simulink model "E040S0_S2_guard_shed_iqcot_20260629"  (R2024b)
settings: Solver=VariableStepAuto  StartTime=0.0  StopTime=0.52e-3  MaxStep=5e-9  RelTol=1e-3
undefined symbols (not defined in the file): A_init, A_lower, A_upper, Cout, DCR_L1, DCR_L2, DCR_L3, DCR_L4, E040_Calibration_Enable, E040_Current_Deadband, E040_Current_Limit_A, E040_Dwell_Time, E040_Fallback_K_T, E040_I_Shed_Low, E040_IL_Sense_Gain1, E040_IL_Sense_Gain2, E040_IL_Sense_Gain3, E040_IL_Sense_Gain4, E040_K_T, E040_LoadStep_Time, E040_Min_Scale, E040_Order_Relock_Window, E040_Post_Reentry_Shed_Delay, E040_Residual_Current_Threshold, E040_Sense_Confidence, E040_Severe_Overshoot_Band, E040_T_Trim_Max, E040_TonDiff_Enable, E040_V_Error_Budget, E040_V_Error_Hard_Limit, E040_Variant_Mode, E040_Vref, ESR_C, IdealIQCOT_Enable, IL_adc_counts_per_A, IL_pk_limit_adc_neg, IL_pk_limit_adc_pos, Iload_final, Iload_initial, Iph, Iqcot_enable, kappa_cmd, Kiqcot, Kvc_iqcot, L, Lambda0_iqcot, Lambda_m2, rho_cmd, Ri_iqcot, t_load_step, Tblank, Tdead, Tiqcot_leak, Toff_min, Ton_cmd, Ton_iq_max, Ton_iq_min, Ts_ctrl, Tslot, Tss ... (+6)
libraries: simulink x29, spsCurrentMeasurementLib x8, spsMosfetLib x8, spsSeriesRLCBranchLib x5, spsVoltageMeasurementLib x5, spsDCVoltageSourceLib x4, spsControlledCurrentSourceLib x1, spsGroundLib x1, spspowerguiLib x1
(part 1 of 2)
settings Model: Creator=zengruize  LastModifiedBy=zengruize

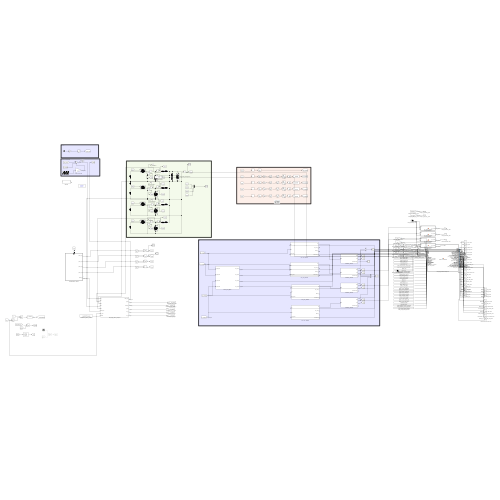
[thumbnail: Simulink's stored preview of the top-level diagram]
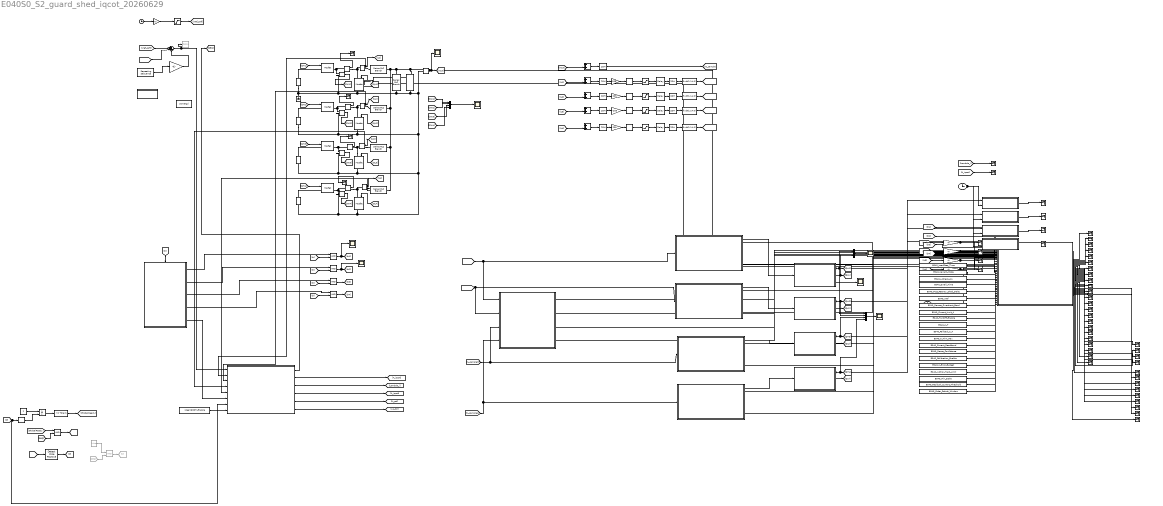
== system E040S0_S2_guard_shed_iqcot_20260629 ==
  note: cot
  note: 输出电压误差比较器
  note: 功率级
  note: 软启动
  note: 采样
  Add{,1..4} (5 alike) : Sum
  Bus Creator : BusCreator  Inputs=4
  Bus Creator1 : BusCreator  Inputs=2
  Bus Creator2 : BusCreator  Inputs=4
  COT_Cell_1Phase1 : Subsystem
  COT_Cell_1Phase2 : Subsystem
  COT_Cell_1Phase3 : Subsystem
  COT_Cell_1Phase4 : Subsystem
  Clock : Clock
  Compare To Constant : simulink/Logic and Bit Operations/Compare To Constant  relop=>=  const=Tblank  OutDataTypeStr=boolean
  Constant : Constant
  Current Measurement{,1..3} (4 alike) : spsCurrentMeasurementLib/Current Measurement  PhasorSimulation=off  OutputType=Complex  PSBequivalent=0
  DC Voltage Source{,1..3} (4 alike) : spsDCVoltageSourceLib/DC Voltage Source  Amplitude=Vin  Measurements=None
  Data Type Conversion{,2..4} (4 alike) : DataTypeConversion  OutDataTypeStr=fixdt(1,14,0)  SaturateOnIntegerOverflow=off  RndMeth=Floor
  Detect Rise Positive : simulink/Logic and Bit Operations/Detect Rise Positive  vinit=0  OutDataTypeStr=boolean
  E040_Calibration_Enable : Constant  Value=E040_Calibration_Enable
  E040_Current_Deadband : Constant  Value=E040_Current_Deadband
  E040_Current_Limit_A : Constant  Value=E040_Current_Limit_A
  E040_Dwell_Time : Constant  Value=E040_Dwell_Time
  E040_Fallback_K_T : Constant  Value=E040_Fallback_K_T
  E040_IL_Sense_Gain_Block1 : Gain  Gain=E040_IL_Sense_Gain1
  E040_IL_Sense_Gain_Block2 : Gain  Gain=E040_IL_Sense_Gain2
  E040_IL_Sense_Gain_Block3 : Gain  Gain=E040_IL_Sense_Gain3
  E040_IL_Sense_Gain_Block4 : Gain  Gain=E040_IL_Sense_Gain4
  E040_IL_Sense_Term{1..4} (4 alike) : Terminator
  E040_I_Shed_Low : Constant  Value=E040_I_Shed_Low
  E040_K_T : Constant  Value=E040_K_T
  E040_LoadCurrentStep : Step  Time=t_load_step  Before=Iload_initial  After=Iload_final  SampleTime=0
  E040_LoadStep_Time : Constant  Value=E040_LoadStep_Time
  E040_Load_Current_Source : spsControlledCurrentSourceLib/Controlled Current Source  Initialize=on  Source_Type=DC  Amplitude=0  Phase=0  Frequency=0  Measurements=None
  E040_Log_Lambda_i_Term : Terminator
  E040_Log_area_int_i_Term : Terminator
  E040_Min_Scale : Constant  Value=E040_Min_Scale
  E040_N_active_Term : Terminator
  E040_Order_Relock_Window : Constant  Value=E040_Order_Relock_Window
  E040_Post_Reentry_Shed_Delay : Constant  Value=E040_Post_Reentry_Shed_Delay
  E040_REQ_accept1_Term : Terminator
  E040_REQ_accept2_Term : Terminator
  E040_REQ_accept3_Term : Terminator
  E040_REQ_accept4_Term : Terminator
  E040_REQ_reject_reason_Term : Terminator
  E040_Residual_Current_Threshold : Constant  Value=E040_Residual_Current_Threshold
  E040_S0_ShedPhaseSupervisor : MATLAB Function  TreatAsAtomicUnit=on
  E040_S0_Supervisor_Clock : Clock
  E040_Sense_Confidence : Constant  Value=E040_Sense_Confidence
  E040_Severe_Overshoot_Band : Constant  Value=E040_Severe_Overshoot_Band
  E040_T_Trim_Max : Constant  Value=E040_T_Trim_Max
  E040_TonActual1 : MATLAB Function  TreatAsAtomicUnit=on  SystemSampleTime=Ts_ctrl
  E040_TonActual1_Term : Terminator
  E040_TonActual2 : MATLAB Function  TreatAsAtomicUnit=on  SystemSampleTime=Ts_ctrl
  E040_TonActual2_Term : Terminator
  E040_TonActual3 : MATLAB Function  TreatAsAtomicUnit=on  SystemSampleTime=Ts_ctrl
  E040_TonActual3_Term : Terminator
  E040_TonActual4 : MATLAB Function  TreatAsAtomicUnit=on  SystemSampleTime=Ts_ctrl
  E040_TonActual4_Term : Terminator
  E040_TonActual_Clock : Clock
  E040_TonDiff_Enable : Constant  Value=E040_TonDiff_Enable
  E040_Ton_trim1_Term : Terminator
  E040_Ton_trim2_Term : Terminator
  E040_Ton_trim3_Term : Terminator
  E040_Ton_trim4_Term : Terminator
  E040_V_Error_Budget : Constant  Value=E040_V_Error_Budget
  E040_V_Error_Hard_Limit : Constant  Value=E040_V_Error_Hard_Limit
  E040_Variant_Mode : Constant  Value=E040_Variant_Mode
  E040_Vref : Constant  Value=E040_Vref
  E040_a_S_enable_after_shed_Term : Terminator
  E040_a_S_mode_Term : Terminator
  E040_active_phase_set_Term : Terminator
  E040_balance_recovery_state_Term : Terminator
  E040_calibration_enable_Term : Terminator
  E040_current_limit_hit_Term : Terminator
  E040_dwell_timer_Term : Terminator
  E040_fallback_count_Term : Terminator
  E040_guard_clamp_count_Term : Terminator
  E040_logical_slot_Term : Terminator
  E040_order_relock_state_Term : Terminator
  E040_order_relock_window_done_Term : Terminator
  E040_phase_add_request_Term : Terminator
  E040_phase_order_error_rate_window_Term : Terminator
  E040_phase_shed_accept_Term : Terminator
  E040_phase_shed_reject_Term : Terminator
  E040_phase_shed_reject_reason_Term : Terminator
  E040_phase_shed_request_Term : Terminator
  E040_physical_phase_selected_Term : Terminator
  E040_post_reentry_shed_delay_timer_Term : Terminator
  E040_protect_state_Term : Terminator
  E040_reentry_state_Term : Terminator
  E040_residual_current_check_Term : Terminator
  E040_residual_current_i_Term : Terminator
  E040_residual_current_threshold_Term : Terminator
  E040_sense_confidence_Term : Terminator
  E040_shed_lockout_state_Term : Terminator
  E040_shed_state_Term : Terminator
  From31 : From  Commented=on  GotoTag=REQ
  Gain : Gain  Gain=Vo_ref / Tss
  Gain11 : Gain  Gain=205
  Gain12 : Gain  Gain=-205
  Gain13 : Gain  Gain=205
  Gain9 : Gain  Gain=-205
  GateDriver_1Phase1 : Subsystem
  GateDriver_1Phase2 : Subsystem
  GateDriver_1Phase3 : Subsystem
  GateDriver_1Phase4 : Subsystem
  Goto26 : Goto  Commented=on  GotoTag=tr
  Ground : spsGroundLib/Ground  LConnTagsString=a
  IHS_Terminator{1..4} (4 alike) : Terminator
  IL_Measurement{1..4} (4 alike) : spsCurrentMeasurementLib/Current Measurement  PhasorSimulation=off  OutputType=Complex  PSBequivalent=0
  IQCOT_Ton_Adapter : Subsystem
  IdealIQCOT_Enable_Constant : Constant  Value=IdealIQCOT_Enable
  Ideal_Digital_IQCOT_Request : Subsystem
  Integrator : Integrator  ExternalReset=rising
  Logical Operator{,1..4} (5 alike) : Logic  AllPortsSameDT=off  OutDataTypeStr=boolean
  Logical Operator5 : Logic  Commented=on  AllPortsSameDT=off  OutDataTypeStr=boolean
  Memory : Memory
  Mosfet{,1..3} (4 alike) : spsMosfetLib/Mosfet  Ron=Ron_HS  Lon=0  Rd=Rd_body  Vfd=Vfd_body  IC=0  Rs=Rs_snubber  Cs=Cs_snubber  Measurements=on
  Mosfet{4..7} (4 alike) : spsMosfetLib/Mosfet  Ron=Ron_LS  Lon=0  Rd=Rd_body  Vfd=Vfd_body  IC=0  Rs=Rs_snubber  Cs=Cs_snubber  Measurements=on
  OnDelay : Subsystem
  PhaseScheduler_4Phase : Subsystem  TreatAsAtomicUnit=on
  Pulse Generator : DiscretePulseGenerator  Commented=on  PulseType=Time based  Period=Tblank  PulseWidth=5
  Quantizer{1..4} (4 alike) : Quantizer  QuantizationInterval=1
  Relay : Relay  Commented=through  OnSwitchValue=Vhys/2  OffSwitchValue=-Vhys/2
  Saturation{,1,3..4} (4 alike) : Saturate  UpperLimit=8191  LowerLimit=-8191
  Saturation2 : Saturate  UpperLimit=Vo_ref  LowerLimit=0
  Scope{,1..6} (7 alike) : Scope
  Series RLC Branch : spsSeriesRLCBranchLib/Series RLC Branch  LConnTagsString=__new0  RConnTagsString=__new0  BranchType=RL  Resistance=DCR_L1  Inductance=L  SetiL0=off  InitialCurrent=0  Capacitance=1e-6  Setx0=off  InitialVoltage=0  Measurements=None
  Series RLC Branch1 : spsSeriesRLCBranchLib/Series RLC Branch  LConnTagsString=__new0  RConnTagsString=__new0  BranchType=RL  Resistance=DCR_L2  Inductance=L  SetiL0=off  InitialCurrent=0  Capacitance=1e-6  Setx0=off  InitialVoltage=0  Measurements=None
  Series RLC Branch2 : spsSeriesRLCBranchLib/Series RLC Branch  LConnTagsString=__new0  RConnTagsString=__new0  BranchType=RL  Resistance=DCR_L3  Inductance=L  SetiL0=off  InitialCurrent=0  Capacitance=1e-6  Setx0=off  InitialVoltage=0  Measurements=None
  Series RLC Branch3 : spsSeriesRLCBranchLib/Series RLC Branch  LConnTagsString=__new0  RConnTagsString=__new0  BranchType=RL  Resistance=DCR_L4  Inductance=L  SetiL0=off  InitialCurrent=0  Capacitance=1e-6  Setx0=off  InitialVoltage=0  Measurements=None
  Series RLC Branch4 : spsSeriesRLCBranchLib/Series RLC Branch  LConnTagsString=__new0  RConnTagsString=__new0  BranchType=RC  Resistance=ESR_C  Inductance=1e-3  SetiL0=off  InitialCurrent=0  Capacitance=Cout  Setx0=on  InitialVoltage=Vo_ref  Measurements=None
  Sum : Sum  Inputs=|+--
  Transport Delay{1..4} (4 alike) : TransportDelay  DelayTime=5/25000000
  VCOT_Ramp_Gain : Gain  Gain=Vcot_ramp_enable * Vcot_ramp_amp
  VCOT_Ramp_Unit : simulink/Sources/Repeating Sequence  rep_seq_t=[0 Tslot]  rep_seq_y=[0 1]
  Voltage Measurement{,1..4} (5 alike) : spsVoltageMeasurementLib/Voltage Measurement  PhasorSimulation=off  OutputType=Complex  PSBequivalent=0
  Zero-Order Hold{1..4,19..23} (9 alike) : ZeroOrderHold  SampleTime=1/25000000
  powergui : spspowerguiLib/powergui  Priority=1  SimulationMode=Discrete  SampleTime=2e-9  frequency=60  Iterations=50  frequencyindice=0  Pbase=100e6  ErrMax=1e-4  UnitsV=kV  UnitsW=MW  buscounter=0  FunctionMessages=off  echomessages=off  EnableUseOfTLC=off  CurrentSourceSwitches=off  DisableSnubberDevices=off  DisableRonSwitches=off  DisableVfSwitches=off  DisplayEquations=off  AutomaticDiscreteSolvers=off  SolverType=Tustin/Backward Euler (TBE)  Interpol=off  ExternalGateDelay=off  methode=off  Ts=100  x0status=blocks  SPID=on  SwTol=0  HookPort=off  NonlinearTolerance=1e-4  nMaxIteration=100  ContinueOnMaxIteration=off  RestoreLinks=warning  ResistiveCurrentMeasurement=off  Frange=[0:2:500]  Ylog=off  Xlog=on  ShowGrid=off  save=off  variable=ZData  structure=0  ZoomFFT=off  StartTime=0.0  cycles=1  DisplayStyle=1  fundamental=60  FreqAxis=off  MaxFrequency=1000  frequencyindicesteady=1  RmsSteady=1  display=off
  wires:
  [QH1] -> Mosfet/1
  [QH4] -> Mosfet3/1
  [QH2] -> Mosfet1/1
  [QH3] -> Mosfet2/1
  [QL1] -> Mosfet4/1
  [QL2] -> Mosfet5/1
  [QL3] -> Mosfet6/1
  [QL4] -> Mosfet7/1
  Voltage Measurement2/1 -> [SW2]  "SW2"
  Voltage Measurement3/1 -> [SW3]  "SW3"
  Voltage Measurement1/1 -> [SW1]  "SW1"
  Voltage Measurement4/1 -> [SW4]  "SW4"
  GateDriver_1Phase1/1(QHi) -> Bus Creator1/1, [QH1], Bus Creator2/1, E040_TonActual1/1(qh)  "QH1"
  GateDriver_1Phase2/1(QHi) -> Bus Creator2/2, [QH2], E040_TonActual2/1(qh)  "QH2"
  GateDriver_1Phase3/1(QHi) -> Bus Creator2/3, [QH3], E040_TonActual3/1(qh)  "QH3"
  GateDriver_1Phase4/1(QHi) -> Bus Creator2/4, [QH4], E040_TonActual4/1(qh)  "QH4"
  GateDriver_1Phase1/2(QLi) -> Bus Creator1/2, [QL1]  "QL1"
  GateDriver_1Phase2/2(QLi) -> [QL2]  "QL2"
  GateDriver_1Phase3/2(QLi) -> [QL3]  "QL3"
  GateDriver_1Phase4/2(QLi) -> [QL4]  "QL4"
  COT_Cell_1Phase1/1(Qi) -> GateDriver_1Phase1/1(Qi)
  COT_Cell_1Phase2/1(Qi) -> GateDriver_1Phase2/1(Qi)
  COT_Cell_1Phase3/1(Qi) -> GateDriver_1Phase3/1(Qi)
  COT_Cell_1Phase4/1(Qi) -> GateDriver_1Phase4/1(Qi)
  GateDriver_1Phase1/3(ShootThrough_i) -> Scope1/1
  Bus Creator/1 -> Scope2/1
  [SW1] -> Bus Creator/1
  [SW2] -> Bus Creator/2
  [SW3] -> Bus Creator/3
  [SW4] -> Bus Creator/4
  Bus Creator1/1 -> Scope3/1
  Saturation2/1 -> [Vref_soft]
  Gain/1 -> Saturation2/1
  Clock/1 -> Gain/1
  Voltage Measurement/1 -> Scope/1, [Vout], E040_S0_ShedPhaseSupervisor/13(vout)  "Vout"
  [Vref_soft] -> Sum/1
  [Vo_sample] -> Sum/2
  Sum/1 -> Ideal_Digital_IQCOT_Request/1(e_v), Relay/1  "e_v"
  Constant/1 -> Integrator/1
  Integrator/1 -> Compare To Constant/1
  Compare To Constant/1 -> [GlobalReady]  "Allow"
  [GlobalReady] -> Logical Operator/1
  [REQ] -> Logical Operator/2
  Logical Operator/1 -> [Allow]
  [Allow] -> Detect Rise Positive/1
  Detect Rise Positive/1 -> [tr]
  [tr] -> PhaseScheduler_4Phase/Trigger  "tr"
  PhaseScheduler_4Phase/1(phase_en1) -> Logical Operator1/1
  [tr] -> Logical Operator1/2
  PhaseScheduler_4Phase/2(phase_en2) -> Logical Operator2/1
  [tr] -> Logical Operator2/2
  PhaseScheduler_4Phase/3(phase_en3) -> Logical Operator3/1
  [tr] -> Logical Operator3/2
  PhaseScheduler_4Phase/4(phase_en4) -> Logical Operator4/1
  [tr] -> Logical Operator4/2
  Logical Operator1/1 -> Scope4/1, [tr1]  "tr1"
  Logical Operator2/1 -> Scope5/1, [tr2]  "tr2"
  Logical Operator3/1 -> [tr3]  "tr3"
  Logical Operator4/1 -> [tr4]  "tr4"
  [IL_sample1] -> COT_Cell_1Phase1/2(ILi), IQCOT_Ton_Adapter/1(IL_sample1)  "IL_sample1"
  [IL_sample2] -> IQCOT_Ton_Adapter/2(IL_sample2), COT_Cell_1Phase2/2(ILi)  "IL_sample2"
  [IL_sample3] -> IQCOT_Ton_Adapter/3(IL_sample3), COT_Cell_1Phase3/2(ILi)  "IL_sample3"
  [IL_sample4] -> IQCOT_Ton_Adapter/4(IL_sample4), COT_Cell_1Phase4/2(ILi)  "IL_sample4"
  [tr] -> Memory/1, Ideal_Digital_IQCOT_Request/7(tr_reset)  "tr_reset"
  Memory/1 -> Integrator/2
  Logical Operator5/1 -> Goto26/1
  Pulse Generator/1 -> Logical Operator5/1
  From31/1 -> Logical Operator5/2
  Bus Creator2/1 -> Scope6/1
  IL_Measurement1/1 -> [IL1], Ideal_Digital_IQCOT_Request/2(IL1)  "IL1"
  IL_Measurement2/1 -> [IL2], Ideal_Digital_IQCOT_Request/3(IL2)  "IL2"
  IL_Measurement3/1 -> [IL3], Ideal_Digital_IQCOT_Request/4(IL3)  "IL3"
  IL_Measurement4/1 -> [IL4], Ideal_Digital_IQCOT_Request/5(IL4)  "IL4"
  Current Measurement/1 -> IHS_Terminator1/1
  Current Measurement1/1 -> IHS_Terminator2/1
  Current Measurement2/1 -> IHS_Terminator3/1
  Current Measurement3/1 -> IHS_Terminator4/1
  Zero-Order Hold23/1 -> Gain13/1
  Zero-Order Hold20/1 -> Gain9/1
  Zero-Order Hold3/1 -> Data Type Conversion3/1
  Zero-Order Hold4/1 -> Data Type Conversion2/1
  Saturation4/1 -> Transport Delay4/1
  Zero-Order Hold1/1 -> Data Type Conversion/1
  [IL3] -> Add3/2
  Add3/1 -> Zero-Order Hold22/1
  Quantizer1/1 -> Saturation/1
  Quantizer4/1 -> Saturation4/1
  Gain12/1 -> Quantizer3/1
  [IL4] -> Add4/2
  Add/1 -> Zero-Order Hold19/1
  Data Type Conversion/1 -> [IL_sample1]
  Data Type Conversion2/1 -> [IL_sample4]
  Add4/1 -> Zero-Order Hold23/1
  Transport Delay3/1 -> Zero-Order Hold3/1
  Saturation3/1 -> Transport Delay3/1
  Add1/1 -> Zero-Order Hold20/1
  [IL1] -> Add1/2
  Transport Delay4/1 -> Zero-Order Hold4/1
  Zero-Order Hold21/1 -> Gain11/1
  Data Type Conversion3/1 -> [IL_sample3]
  Gain9/1 -> Quantizer1/1
  Gain11/1 -> Quantizer2/1
  Saturation/1 -> Transport Delay1/1
  [IL2] -> Add2/2
  Transport Delay2/1 -> Zero-Order Hold2/1
  Zero-Order Hold19/1 -> [Vo_sample]
  Gain13/1 -> Quantizer4/1
  Quantizer3/1 -> Saturation3/1
  Data Type Conversion4/1 -> [IL_sample2]
  Zero-Order Hold2/1 -> Data Type Conversion4/1
  Add2/1 -> Zero-Order Hold21/1
  Transport Delay1/1 -> Zero-Order Hold1/1
  [Vout] -> Add/2
  Saturation1/1 -> Transport Delay2/1
  Zero-Order Hold22/1 -> Gain12/1
  Quantizer2/1 -> Saturation1/1
  VCOT_Ramp_Unit/1 -> VCOT_Ramp_Gain/1
  VCOT_Ramp_Gain/1 -> Sum/3  "Vcot_ramp"
  PhaseScheduler_4Phase/5(phase_idx) -> Ideal_Digital_IQCOT_Request/6(phase_idx)  "phase_idx"
  IdealIQCOT_Enable_Constant/1 -> Ideal_Digital_IQCOT_Request/8(enable)
  Ideal_Digital_IQCOT_Request/1(REQ_iqcot) -> [REQ]  "REQ_iqcot"
  Ideal_Digital_IQCOT_Request/2(A_iqcot) -> [A_iqcot]  "A_iqcot"
  Ideal_Digital_IQCOT_Request/3(Lambda_i) -> [Lambda_i]  "Lambda_i"
  Ideal_Digital_IQCOT_Request/4(h_iqcot) -> [h_iqcot]  "h_iqcot"
  Ideal_Digital_IQCOT_Request/5(IL_sel) -> [IL_sel]  "IL_sel"
  Ideal_Digital_IQCOT_Request/6(vc_ctrl) -> [vc_ctrl]  "vc_ctrl"
  E040_LoadCurrentStep/1 -> E040_Load_Current_Source/1, E040_S0_ShedPhaseSupervisor/14(iload)  "Iload"
  [IL1] -> E040_IL_Sense_Gain_Block1/1
  E040_IL_Sense_Gain_Block1/1 -> E040_IL_Sense_Term1/1, E040_S0_ShedPhaseSupervisor/9(il1)  "IL_sense1"
  [IL2] -> E040_IL_Sense_Gain_Block2/1
  E040_IL_Sense_Gain_Block2/1 -> E040_IL_Sense_Term2/1, E040_S0_ShedPhaseSupervisor/10(il2)  "IL_sense2"
  [IL3] -> E040_IL_Sense_Gain_Block3/1
  E040_IL_Sense_Gain_Block3/1 -> E040_IL_Sense_Term3/1, E040_S0_ShedPhaseSupervisor/11(il3)  "IL_sense3"
  [IL4] -> E040_IL_Sense_Gain_Block4/1
  E040_IL_Sense_Gain_Block4/1 -> E040_IL_Sense_Term4/1, E040_S0_ShedPhaseSupervisor/12(il4)  "IL_sense4"
  [tr1] -> E040_S0_ShedPhaseSupervisor/1(req1)  "REQ_raw1"
  E040_S0_ShedPhaseSupervisor/1(req1o) -> COT_Cell_1Phase1/1(tri)  "REQ1"
  IQCOT_Ton_Adapter/1(Ton_iqcot1) -> E040_S0_ShedPhaseSupervisor/5(ton1)  "Ton_raw1"
  E040_S0_ShedPhaseSupervisor/5(ton1o) -> COT_Cell_1Phase1/3(Ton_iqcot1)  "Ton_cmd1"
  [tr2] -> E040_S0_ShedPhaseSupervisor/2(req2)  "REQ_raw2"
  E040_S0_ShedPhaseSupervisor/2(req2o) -> COT_Cell_1Phase2/1(tri)  "REQ2"
  IQCOT_Ton_Adapter/2(Ton_iqcot2) -> E040_S0_ShedPhaseSupervisor/6(ton2)  "Ton_raw2"
  E040_S0_ShedPhaseSupervisor/6(ton2o) -> COT_Cell_1Phase2/3(Ton_iqcot2)  "Ton_cmd2"
  [tr3] -> E040_S0_ShedPhaseSupervisor/3(req3)  "REQ_raw3"
  E040_S0_ShedPhaseSupervisor/3(req3o) -> COT_Cell_1Phase3/1(tri)  "REQ3"
  IQCOT_Ton_Adapter/3(Ton_iqcot3) -> E040_S0_ShedPhaseSupervisor/7(ton3)  "Ton_raw3"
  E040_S0_ShedPhaseSupervisor/7(ton3o) -> COT_Cell_1Phase3/3(Ton_iqcot3)  "Ton_cmd3"
  [tr4] -> E040_S0_ShedPhaseSupervisor/4(req4)  "REQ_raw4"
  E040_S0_ShedPhaseSupervisor/4(req4o) -> COT_Cell_1Phase4/1(tri)  "REQ4"
  IQCOT_Ton_Adapter/4(Ton_iqcot4) -> E040_S0_ShedPhaseSupervisor/8(ton4)  "Ton_raw4"
  E040_S0_ShedPhaseSupervisor/8(ton4o) -> COT_Cell_1Phase4/3(Ton_iqcot4)  "Ton_cmd4"
  E040_S0_Supervisor_Clock/1 -> E040_S0_ShedPhaseSupervisor/15(t)
  E040_LoadStep_Time/1 -> E040_S0_ShedPhaseSupervisor/16(t_step)
  E040_Variant_Mode/1 -> E040_S0_ShedPhaseSupervisor/17(variant_mode)
  E040_I_Shed_Low/1 -> E040_S0_ShedPhaseSupervisor/18(I_shed_low)
  E040_Dwell_Time/1 -> E040_S0_ShedPhaseSupervisor/19(dwell_time)
  E040_Post_Reentry_Shed_Delay/1 -> E040_S0_ShedPhaseSupervisor/20(post_reentry_shed_delay)
  E040_Vref/1 -> E040_S0_ShedPhaseSupervisor/21(Vref)
  E040_Severe_Overshoot_Band/1 -> E040_S0_ShedPhaseSupervisor/22(severe_overshoot_band)
  E040_Current_Limit_A/1 -> E040_S0_ShedPhaseSupervisor/23(current_limit_A)
  E040_TonDiff_Enable/1 -> E040_S0_ShedPhaseSupervisor/24(TonDiff_enable)
  E040_K_T/1 -> E040_S0_ShedPhaseSupervisor/25(K_T)
  E040_Fallback_K_T/1 -> E040_S0_ShedPhaseSupervisor/26(fallback_K_T)
  E040_T_Trim_Max/1 -> E040_S0_ShedPhaseSupervisor/27(T_trim_Max)
  E040_Current_Deadband/1 -> E040_S0_ShedPhaseSupervisor/28(current_deadband)
  E040_Sense_Confidence/1 -> E040_S0_ShedPhaseSupervisor/29(sense_confidence)
  E040_Calibration_Enable/1 -> E040_S0_ShedPhaseSupervisor/30(calibration_enable)
  E040_V_Error_Budget/1 -> E040_S0_ShedPhaseSupervisor/31(Verr_budget)
  E040_V_Error_Hard_Limit/1 -> E040_S0_ShedPhaseSupervisor/32(Verr_hard)
  E040_Min_Scale/1 -> E040_S0_ShedPhaseSupervisor/33(min_scale)
  E040_Residual_Current_Threshold/1 -> E040_S0_ShedPhaseSupervisor/34(residual_current_threshold)
  E040_Order_Relock_Window/1 -> E040_S0_ShedPhaseSupervisor/35(order_relock_window)
  E040_S0_ShedPhaseSupervisor/9(active_phase_set) -> E040_active_phase_set_Term/1  "active_phase_set"
  E040_S0_ShedPhaseSupervisor/10(N_active) -> E040_N_active_Term/1  "N_active"
  E040_S0_ShedPhaseSupervisor/11(phase_shed_request) -> E040_phase_shed_request_Term/1  "phase_shed_request"
  E040_S0_ShedPhaseSupervisor/12(phase_shed_accept) -> E040_phase_shed_accept_Term/1  "phase_shed_accept"
  E040_S0_ShedPhaseSupervisor/13(phase_shed_reject) -> E040_phase_shed_reject_Term/1  "phase_shed_reject"
  E040_S0_ShedPhaseSupervisor/14(phase_add_request) -> E040_phase_add_request_Term/1  "phase_add_request"
  E040_S0_ShedPhaseSupervisor/15(shed_state) -> E040_shed_state_Term/1  "shed_state"
  E040_S0_ShedPhaseSupervisor/16(shed_lockout_state) -> E040_shed_lockout_state_Term/1  "shed_lockout_state"
  E040_S0_ShedPhaseSupervisor/17(residual_current_i) -> E040_residual_current_i_Term/1  "residual_current_i"
  E040_S0_ShedPhaseSupervisor/18(residual_current_threshold_o) -> E040_residual_current_threshold_Term/1  "residual_current_threshold"
  E040_S0_ShedPhaseSupervisor/19(residual_current_check) -> E040_residual_current_check_Term/1  "residual_current_check"
  E040_S0_ShedPhaseSupervisor/20(dwell_timer) -> E040_dwell_timer_Term/1  "dwell_timer"
  E040_S0_ShedPhaseSupervisor/21(post_reentry_shed_delay_timer) -> E040_post_reentry_shed_delay_timer_Term/1  "post_reentry_shed_delay_timer"
  E040_S0_ShedPhaseSupervisor/22(protect_state) -> E040_protect_state_Term/1  "protect_state"
  E040_S0_ShedPhaseSupervisor/23(reentry_state) -> E040_reentry_state_Term/1  "reentry_state"
  E040_S0_ShedPhaseSupervisor/24(balance_recovery_state) -> E040_balance_recovery_state_Term/1  "balance_recovery_state"
  E040_S0_ShedPhaseSupervisor/25(sense_confidence_o) -> E040_sense_confidence_Term/1  "sense_confidence"
  E040_S0_ShedPhaseSupervisor/26(calibration_enable_o) -> E040_calibration_enable_Term/1  "calibration_enable"
  E040_S0_ShedPhaseSupervisor/27(a_S_mode) -> E040_a_S_mode_Term/1  "a_S_mode"
  E040_S0_ShedPhaseSupervisor/28(fallback_count_o) -> E040_fallback_count_Term/1  "fallback_count"
  E040_S0_ShedPhaseSupervisor/29(guard_clamp_count_o) -> E040_guard_clamp_count_Term/1  "guard_clamp_count"
  E040_S0_ShedPhaseSupervisor/30(trim1) -> E040_Ton_trim1_Term/1  "Ton_trim1"
  E040_S0_ShedPhaseSupervisor/31(trim2) -> E040_Ton_trim2_Term/1  "Ton_trim2"
  E040_S0_ShedPhaseSupervisor/32(trim3) -> E040_Ton_trim3_Term/1  "Ton_trim3"
  E040_S0_ShedPhaseSupervisor/33(trim4) -> E040_Ton_trim4_Term/1  "Ton_trim4"
  E040_S0_ShedPhaseSupervisor/34(REQ_accept1) -> E040_REQ_accept1_Term/1  "REQ_accept1"
  E040_S0_ShedPhaseSupervisor/35(REQ_accept2) -> E040_REQ_accept2_Term/1  "REQ_accept2"
  E040_S0_ShedPhaseSupervisor/36(REQ_accept3) -> E040_REQ_accept3_Term/1  "REQ_accept3"
  E040_S0_ShedPhaseSupervisor/37(REQ_accept4) -> E040_REQ_accept4_Term/1  "REQ_accept4"
  E040_S0_ShedPhaseSupervisor/38(REQ_reject_reason) -> E040_REQ_reject_reason_Term/1  "REQ_reject_reason"
  E040_S0_ShedPhaseSupervisor/39(logical_slot) -> E040_logical_slot_Term/1  "logical_slot"
  E040_S0_ShedPhaseSupervisor/40(physical_phase_selected) -> E040_physical_phase_selected_Term/1  "physical_phase_selected"
  E040_S0_ShedPhaseSupervisor/41(phase_shed_reject_reason) -> E040_phase_shed_reject_reason_Term/1  "phase_shed_reject_reason"
  E040_S0_ShedPhaseSupervisor/42(order_relock_state) -> E040_order_relock_state_Term/1  "order_relock_state"
  E040_S0_ShedPhaseSupervisor/43(order_relock_window_done) -> E040_order_relock_window_done_Term/1  "order_relock_window_done"
  E040_S0_ShedPhaseSupervisor/44(phase_order_error_rate_window) -> E040_phase_order_error_rate_window_Term/1  "phase_order_error_rate_window"
  E040_S0_ShedPhaseSupervisor/45(a_S_enable_after_shed) -> E040_a_S_enable_after_shed_Term/1  "a_S_enable_after_shed"
  E040_S0_ShedPhaseSupervisor/46(current_limit_hit) -> E040_current_limit_hit_Term/1  "current_limit_hit"
  [Lambda_i] -> E040_Log_Lambda_i_Term/1  "Lambda_i"
  [A_iqcot] -> E040_Log_area_int_i_Term/1  "area_int_i"
  E040_TonActual_Clock/1 -> E040_TonActual1/2(t), E040_TonActual2/2(t), E040_TonActual3/2(t), E040_TonActual4/2(t)
  E040_TonActual1/1(Ton_actual) -> E040_TonActual1_Term/1  "Ton_actual1"
  E040_TonActual2/1(Ton_actual) -> E040_TonActual2_Term/1  "Ton_actual2"
  E040_TonActual3/1(Ton_actual) -> E040_TonActual3_Term/1  "Ton_actual3"
  E040_TonActual4/1(Ton_actual) -> E040_TonActual4_Term/1  "Ton_actual4"
  connections:
  DC Voltage Source/LConn1 -- Voltage Measurement1/LConn2 -- Mosfet7/RConn1 -- Voltage Measurement4/LConn2 -- DC Voltage Source3/LConn1 -- Mosfet6/RConn1 -- Voltage Measurement3/LConn2 -- DC Voltage Source2/LConn1 -- DC Voltage Source1/LConn1 -- Voltage Measurement2/LConn2 -- Mosfet5/RConn1 -- Voltage Measurement/LConn2 -- E040_Load_Current_Source/RConn1 -- Series RLC Branch4/RConn1 -- Mosfet4/RConn1 -- Ground/LConn1
  Mosfet/LConn1 -- DC Voltage Source/RConn1
  DC Voltage Source1/RConn1 -- Mosfet1/LConn1
  Mosfet1/RConn1 -- Current Measurement1/LConn1 -- Voltage Measurement2/LConn1
  DC Voltage Source2/RConn1 -- Mosfet2/LConn1
  Mosfet2/RConn1 -- Current Measurement2/LConn1 -- Voltage Measurement3/LConn1
  DC Voltage Source3/RConn1 -- Mosfet3/LConn1
  Series RLC Branch/RConn1 -- Series RLC Branch3/RConn1 -- Series RLC Branch2/RConn1 -- Series RLC Branch1/RConn1 -- Voltage Measurement/LConn1 -- E040_Load_Current_Source/LConn1 -- Series RLC Branch4/LConn1
  Mosfet/RConn1 -- Current Measurement/LConn1 -- Voltage Measurement1/LConn1
  Mosfet3/RConn1 -- Current Measurement3/LConn1 -- Voltage Measurement4/LConn1
  Current Measurement/RConn1 -- Mosfet4/LConn1 -- IL_Measurement1/LConn1
  IL_Measurement1/RConn1 -- Series RLC Branch/LConn1
  Current Measurement1/RConn1 -- Mosfet5/LConn1 -- IL_Measurement2/LConn1
  IL_Measurement2/RConn1 -- Series RLC Branch1/LConn1
  Mosfet6/LConn1 -- Current Measurement2/RConn1 -- IL_Measurement3/LConn1
  IL_Measurement3/RConn1 -- Series RLC Branch2/LConn1
  Current Measurement3/RConn1 -- Mosfet7/LConn1 -- IL_Measurement4/LConn1
  IL_Measurement4/RConn1 -- Series RLC Branch3/LConn1

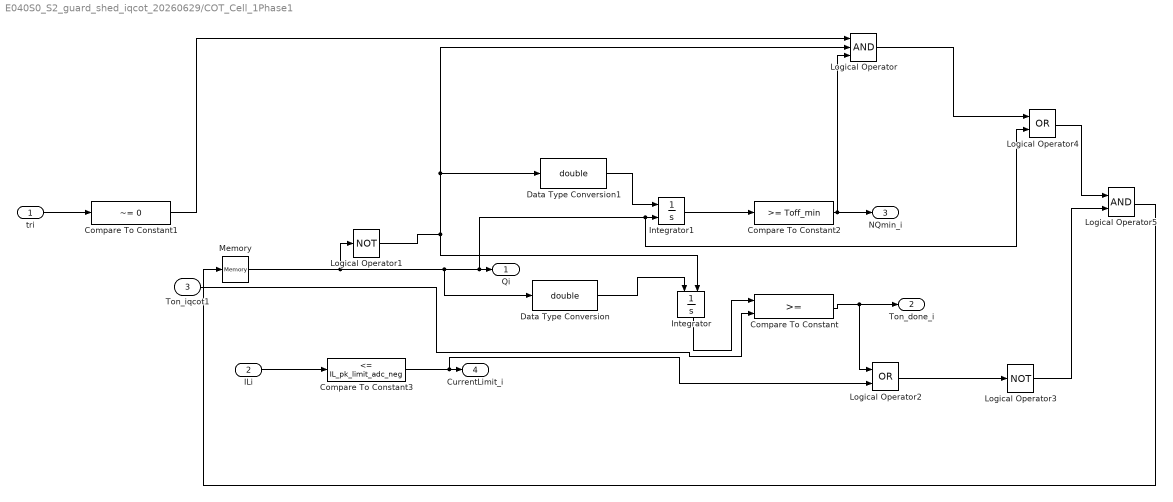
== system E040S0_S2_guard_shed_iqcot_20260629/COT_Cell_1Phase1 ==
  tri : Inport
  ILi : Inport  Port=2
  Ton_iqcot1 : Inport  Port=3
  Compare To Constant : RelationalOperator  OutDataTypeStr=boolean  RndMeth=Simplest  InputSameDT=off
  Compare To Constant1 : simulink/Logic and Bit Operations/Compare To Constant  relop=~=  const=0  OutDataTypeStr=boolean
  Compare To Constant2 : simulink/Logic and Bit Operations/Compare To Constant  relop=>=  const=Toff_min  OutDataTypeStr=boolean
  Compare To Constant3 : simulink/Logic and Bit Operations/Compare To Constant  relop=<=  const=IL_pk_limit_adc_neg  OutDataTypeStr=boolean
  Data Type Conversion : DataTypeConversion  OutDataTypeStr=double  SaturateOnIntegerOverflow=off  RndMeth=Floor
  Data Type Conversion1 : DataTypeConversion  OutDataTypeStr=double  SaturateOnIntegerOverflow=off  RndMeth=Floor
  Integrator : Integrator  ExternalReset=level
  Integrator1 : Integrator  ExternalReset=level  InitialCondition=Toff_min
  Logical Operator : Logic  Inputs=3  AllPortsSameDT=off  OutDataTypeStr=boolean
  Logical Operator1 : Logic  Operator=NOT  AllPortsSameDT=off  OutDataTypeStr=boolean
  Logical Operator2 : Logic  Operator=OR  AllPortsSameDT=off  OutDataTypeStr=boolean
  Logical Operator3 : Logic  Operator=NOT  Inputs=3  AllPortsSameDT=off  OutDataTypeStr=boolean
  Logical Operator4 : Logic  Operator=OR  AllPortsSameDT=off  OutDataTypeStr=boolean
  Logical Operator5 : Logic  AllPortsSameDT=off  OutDataTypeStr=boolean
  Memory : Memory
  Qi : Outport
  Ton_done_i : Outport  Port=2
  NQmin_i : Outport  Port=3
  CurrentLimit_i : Outport  Port=4
  wires:
  Compare To Constant/1 -> Logical Operator2/1, Ton_done_i/1
  tri/1 -> Compare To Constant1/1
  Compare To Constant1/1 -> Logical Operator/1
  Memory/1 -> Logical Operator1/1, Data Type Conversion/1, Logical Operator4/2, Integrator1/2, Qi/1
  Logical Operator1/1 -> Data Type Conversion1/1, Logical Operator/2, Integrator/2
  Data Type Conversion/1 -> Integrator/1
  Integrator/1 -> Compare To Constant/1
  Data Type Conversion1/1 -> Integrator1/1
  Integrator1/1 -> Compare To Constant2/1
  Compare To Constant2/1 -> Logical Operator/3, NQmin_i/1
  ILi/1 -> Compare To Constant3/1
  Compare To Constant3/1 -> Logical Operator2/2, CurrentLimit_i/1
  Logical Operator2/1 -> Logical Operator3/1
  Logical Operator/1 -> Logical Operator4/1
  Logical Operator4/1 -> Logical Operator5/1
  Logical Operator3/1 -> Logical Operator5/2
  Logical Operator5/1 -> Memory/1
  Ton_iqcot1/1 -> Compare To Constant/2

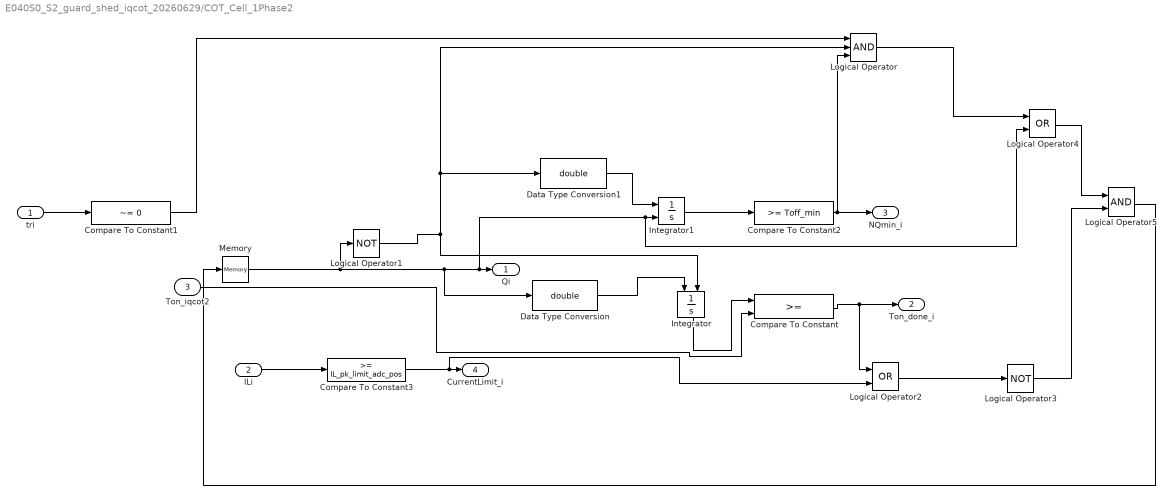
== system E040S0_S2_guard_shed_iqcot_20260629/COT_Cell_1Phase2 ==
  tri : Inport
  ILi : Inport  Port=2
  Ton_iqcot2 : Inport  Port=3
  Compare To Constant : RelationalOperator  OutDataTypeStr=boolean  RndMeth=Simplest  InputSameDT=off
  Compare To Constant1 : simulink/Logic and Bit Operations/Compare To Constant  relop=~=  const=0  OutDataTypeStr=boolean
  Compare To Constant2 : simulink/Logic and Bit Operations/Compare To Constant  relop=>=  const=Toff_min  OutDataTypeStr=boolean
  Compare To Constant3 : simulink/Logic and Bit Operations/Compare To Constant  relop=>=  const=IL_pk_limit_adc_pos  OutDataTypeStr=boolean
  Data Type Conversion : DataTypeConversion  OutDataTypeStr=double  SaturateOnIntegerOverflow=off  RndMeth=Floor
  Data Type Conversion1 : DataTypeConversion  OutDataTypeStr=double  SaturateOnIntegerOverflow=off  RndMeth=Floor
  Integrator : Integrator  ExternalReset=level
  Integrator1 : Integrator  ExternalReset=level  InitialCondition=Toff_min
  Logical Operator : Logic  Inputs=3  AllPortsSameDT=off  OutDataTypeStr=boolean
  Logical Operator1 : Logic  Operator=NOT  AllPortsSameDT=off  OutDataTypeStr=boolean
  Logical Operator2 : Logic  Operator=OR  AllPortsSameDT=off  OutDataTypeStr=boolean
  Logical Operator3 : Logic  Operator=NOT  Inputs=3  AllPortsSameDT=off  OutDataTypeStr=boolean
  Logical Operator4 : Logic  Operator=OR  AllPortsSameDT=off  OutDataTypeStr=boolean
  Logical Operator5 : Logic  AllPortsSameDT=off  OutDataTypeStr=boolean
  Memory : Memory
  Qi : Outport
  Ton_done_i : Outport  Port=2
  NQmin_i : Outport  Port=3
  CurrentLimit_i : Outport  Port=4
  wires:
  Compare To Constant/1 -> Logical Operator2/1, Ton_done_i/1
  tri/1 -> Compare To Constant1/1
  Compare To Constant1/1 -> Logical Operator/1
  Memory/1 -> Logical Operator1/1, Data Type Conversion/1, Logical Operator4/2, Integrator1/2, Qi/1
  Logical Operator1/1 -> Data Type Conversion1/1, Logical Operator/2, Integrator/2
  Data Type Conversion/1 -> Integrator/1
  Integrator/1 -> Compare To Constant/1
  Data Type Conversion1/1 -> Integrator1/1
  Integrator1/1 -> Compare To Constant2/1
  Compare To Constant2/1 -> Logical Operator/3, NQmin_i/1
  ILi/1 -> Compare To Constant3/1
  Compare To Constant3/1 -> Logical Operator2/2, CurrentLimit_i/1
  Logical Operator2/1 -> Logical Operator3/1
  Logical Operator/1 -> Logical Operator4/1
  Logical Operator4/1 -> Logical Operator5/1
  Logical Operator3/1 -> Logical Operator5/2
  Logical Operator5/1 -> Memory/1
  Ton_iqcot2/1 -> Compare To Constant/2

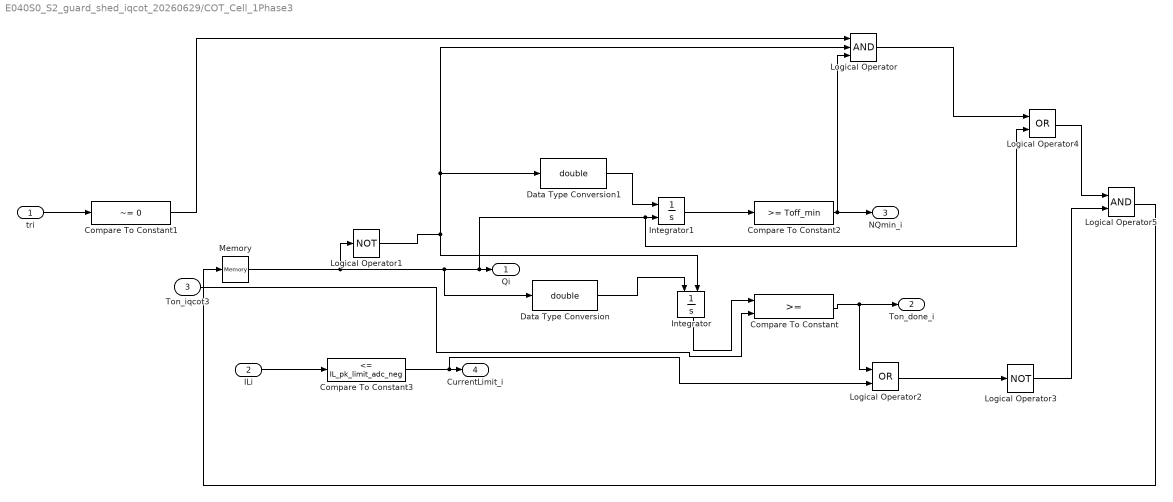
== system E040S0_S2_guard_shed_iqcot_20260629/COT_Cell_1Phase3 ==
  tri : Inport
  ILi : Inport  Port=2
  Ton_iqcot3 : Inport  Port=3
  Compare To Constant : RelationalOperator  OutDataTypeStr=boolean  RndMeth=Simplest  InputSameDT=off
  Compare To Constant1 : simulink/Logic and Bit Operations/Compare To Constant  relop=~=  const=0  OutDataTypeStr=boolean
  Compare To Constant2 : simulink/Logic and Bit Operations/Compare To Constant  relop=>=  const=Toff_min  OutDataTypeStr=boolean
  Compare To Constant3 : simulink/Logic and Bit Operations/Compare To Constant  relop=<=  const=IL_pk_limit_adc_neg  OutDataTypeStr=boolean
  Data Type Conversion : DataTypeConversion  OutDataTypeStr=double  SaturateOnIntegerOverflow=off  RndMeth=Floor
  Data Type Conversion1 : DataTypeConversion  OutDataTypeStr=double  SaturateOnIntegerOverflow=off  RndMeth=Floor
  Integrator : Integrator  ExternalReset=level
  Integrator1 : Integrator  ExternalReset=level  InitialCondition=Toff_min
  Logical Operator : Logic  Inputs=3  AllPortsSameDT=off  OutDataTypeStr=boolean
  Logical Operator1 : Logic  Operator=NOT  AllPortsSameDT=off  OutDataTypeStr=boolean
  Logical Operator2 : Logic  Operator=OR  AllPortsSameDT=off  OutDataTypeStr=boolean
  Logical Operator3 : Logic  Operator=NOT  Inputs=3  AllPortsSameDT=off  OutDataTypeStr=boolean
  Logical Operator4 : Logic  Operator=OR  AllPortsSameDT=off  OutDataTypeStr=boolean
  Logical Operator5 : Logic  AllPortsSameDT=off  OutDataTypeStr=boolean
  Memory : Memory
  Qi : Outport
  Ton_done_i : Outport  Port=2
  NQmin_i : Outport  Port=3
  CurrentLimit_i : Outport  Port=4
  wires:
  Compare To Constant/1 -> Logical Operator2/1, Ton_done_i/1
  tri/1 -> Compare To Constant1/1
  Compare To Constant1/1 -> Logical Operator/1
  Memory/1 -> Logical Operator1/1, Data Type Conversion/1, Logical Operator4/2, Integrator1/2, Qi/1
  Logical Operator1/1 -> Data Type Conversion1/1, Logical Operator/2, Integrator/2
  Data Type Conversion/1 -> Integrator/1
  Integrator/1 -> Compare To Constant/1
  Data Type Conversion1/1 -> Integrator1/1
  Integrator1/1 -> Compare To Constant2/1
  Compare To Constant2/1 -> Logical Operator/3, NQmin_i/1
  ILi/1 -> Compare To Constant3/1
  Compare To Constant3/1 -> Logical Operator2/2, CurrentLimit_i/1
  Logical Operator2/1 -> Logical Operator3/1
  Logical Operator/1 -> Logical Operator4/1
  Logical Operator4/1 -> Logical Operator5/1
  Logical Operator3/1 -> Logical Operator5/2
  Logical Operator5/1 -> Memory/1
  Ton_iqcot3/1 -> Compare To Constant/2

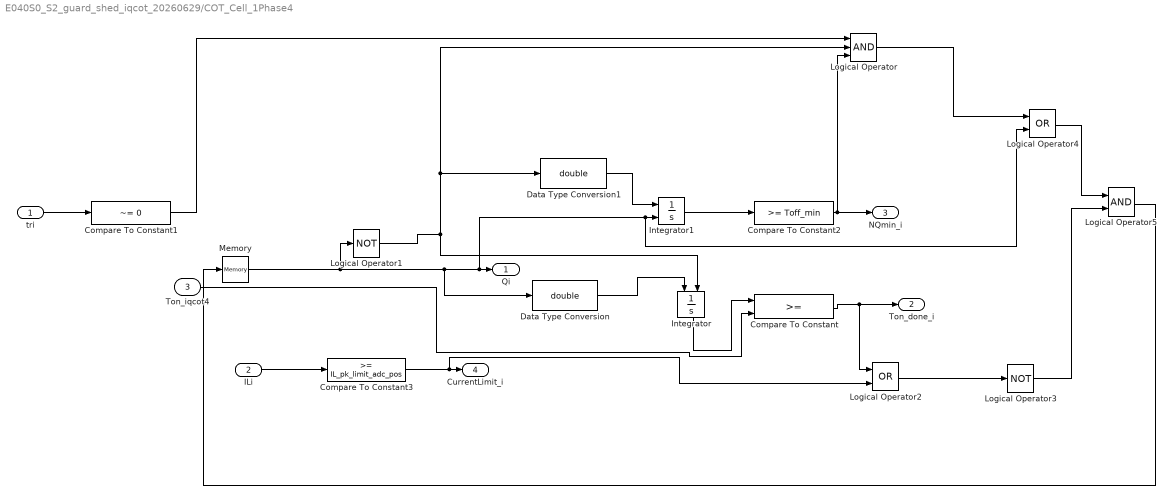
== system E040S0_S2_guard_shed_iqcot_20260629/COT_Cell_1Phase4 ==
  tri : Inport
  ILi : Inport  Port=2
  Ton_iqcot4 : Inport  Port=3
  Compare To Constant : RelationalOperator  OutDataTypeStr=boolean  RndMeth=Simplest  InputSameDT=off
  Compare To Constant1 : simulink/Logic and Bit Operations/Compare To Constant  relop=~=  const=0  OutDataTypeStr=boolean
  Compare To Constant2 : simulink/Logic and Bit Operations/Compare To Constant  relop=>=  const=Toff_min  OutDataTypeStr=boolean
  Compare To Constant3 : simulink/Logic and Bit Operations/Compare To Constant  relop=>=  const=IL_pk_limit_adc_pos  OutDataTypeStr=boolean
  Data Type Conversion : DataTypeConversion  OutDataTypeStr=double  SaturateOnIntegerOverflow=off  RndMeth=Floor
  Data Type Conversion1 : DataTypeConversion  OutDataTypeStr=double  SaturateOnIntegerOverflow=off  RndMeth=Floor
  Integrator : Integrator  ExternalReset=level
  Integrator1 : Integrator  ExternalReset=level  InitialCondition=Toff_min
  Logical Operator : Logic  Inputs=3  AllPortsSameDT=off  OutDataTypeStr=boolean
  Logical Operator1 : Logic  Operator=NOT  AllPortsSameDT=off  OutDataTypeStr=boolean
  Logical Operator2 : Logic  Operator=OR  AllPortsSameDT=off  OutDataTypeStr=boolean
  Logical Operator3 : Logic  Operator=NOT  Inputs=3  AllPortsSameDT=off  OutDataTypeStr=boolean
  Logical Operator4 : Logic  Operator=OR  AllPortsSameDT=off  OutDataTypeStr=boolean
  Logical Operator5 : Logic  AllPortsSameDT=off  OutDataTypeStr=boolean
  Memory : Memory
  Qi : Outport
  Ton_done_i : Outport  Port=2
  NQmin_i : Outport  Port=3
  CurrentLimit_i : Outport  Port=4
  wires:
  Compare To Constant/1 -> Logical Operator2/1, Ton_done_i/1
  tri/1 -> Compare To Constant1/1
  Compare To Constant1/1 -> Logical Operator/1
  Memory/1 -> Logical Operator1/1, Data Type Conversion/1, Logical Operator4/2, Integrator1/2, Qi/1
  Logical Operator1/1 -> Data Type Conversion1/1, Logical Operator/2, Integrator/2
  Data Type Conversion/1 -> Integrator/1
  Integrator/1 -> Compare To Constant/1
  Data Type Conversion1/1 -> Integrator1/1
  Integrator1/1 -> Compare To Constant2/1
  Compare To Constant2/1 -> Logical Operator/3, NQmin_i/1
  ILi/1 -> Compare To Constant3/1
  Compare To Constant3/1 -> Logical Operator2/2, CurrentLimit_i/1
  Logical Operator2/1 -> Logical Operator3/1
  Logical Operator/1 -> Logical Operator4/1
  Logical Operator4/1 -> Logical Operator5/1
  Logical Operator3/1 -> Logical Operator5/2
  Logical Operator5/1 -> Memory/1
  Ton_iqcot4/1 -> Compare To Constant/2

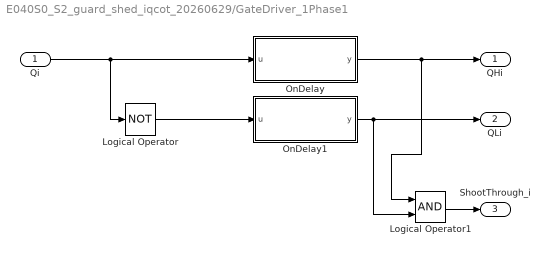
== system E040S0_S2_guard_shed_iqcot_20260629/GateDriver_1Phase1 ==
  Qi : Inport
  Logical Operator : Logic  Operator=NOT  AllPortsSameDT=off  OutDataTypeStr=boolean
  Logical Operator1 : Logic  AllPortsSameDT=off  OutDataTypeStr=boolean
  OnDelay : Subsystem
  OnDelay1 : Subsystem
  QHi : Outport
  QLi : Outport  Port=2
  ShootThrough_i : Outport  Port=3
  wires:
  Qi/1 -> Logical Operator/1, OnDelay/1(u)
  OnDelay/1(y) -> Logical Operator1/1, QHi/1
  Logical Operator/1 -> OnDelay1/1(u)
  OnDelay1/1(y) -> QLi/1, Logical Operator1/2
  Logical Operator1/1 -> ShootThrough_i/1

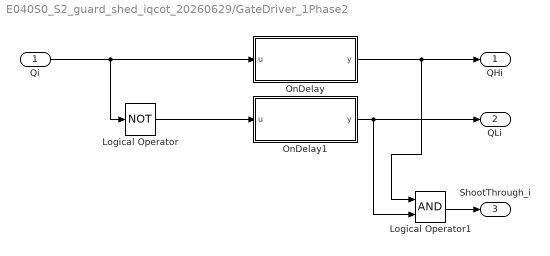
== system E040S0_S2_guard_shed_iqcot_20260629/GateDriver_1Phase2 ==
  Qi : Inport
  Logical Operator : Logic  Operator=NOT  AllPortsSameDT=off  OutDataTypeStr=boolean
  Logical Operator1 : Logic  AllPortsSameDT=off  OutDataTypeStr=boolean
  OnDelay : Subsystem
  OnDelay1 : Subsystem
  QHi : Outport
  QLi : Outport  Port=2
  ShootThrough_i : Outport  Port=3
  wires:
  Qi/1 -> Logical Operator/1, OnDelay/1(u)
  OnDelay/1(y) -> Logical Operator1/1, QHi/1
  Logical Operator/1 -> OnDelay1/1(u)
  OnDelay1/1(y) -> QLi/1, Logical Operator1/2
  Logical Operator1/1 -> ShootThrough_i/1

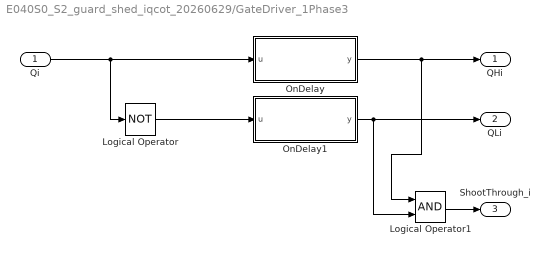
== system E040S0_S2_guard_shed_iqcot_20260629/GateDriver_1Phase3 ==
  Qi : Inport
  Logical Operator : Logic  Operator=NOT  AllPortsSameDT=off  OutDataTypeStr=boolean
  Logical Operator1 : Logic  AllPortsSameDT=off  OutDataTypeStr=boolean
  OnDelay : Subsystem
  OnDelay1 : Subsystem
  QHi : Outport
  QLi : Outport  Port=2
  ShootThrough_i : Outport  Port=3
  wires:
  Qi/1 -> Logical Operator/1, OnDelay/1(u)
  OnDelay/1(y) -> Logical Operator1/1, QHi/1
  Logical Operator/1 -> OnDelay1/1(u)
  OnDelay1/1(y) -> QLi/1, Logical Operator1/2
  Logical Operator1/1 -> ShootThrough_i/1

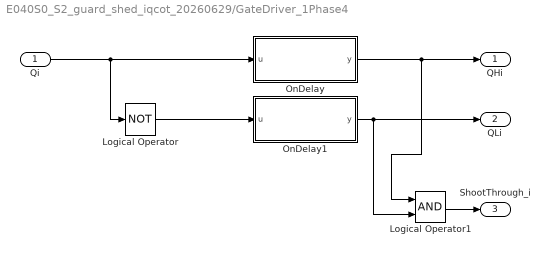
== system E040S0_S2_guard_shed_iqcot_20260629/GateDriver_1Phase4 ==
  Qi : Inport
  Logical Operator : Logic  Operator=NOT  AllPortsSameDT=off  OutDataTypeStr=boolean
  Logical Operator1 : Logic  AllPortsSameDT=off  OutDataTypeStr=boolean
  OnDelay : Subsystem
  OnDelay1 : Subsystem
  QHi : Outport
  QLi : Outport  Port=2
  ShootThrough_i : Outport  Port=3
  wires:
  Qi/1 -> Logical Operator/1, OnDelay/1(u)
  OnDelay/1(y) -> Logical Operator1/1, QHi/1
  Logical Operator/1 -> OnDelay1/1(u)
  OnDelay1/1(y) -> QLi/1, Logical Operator1/2
  Logical Operator1/1 -> ShootThrough_i/1

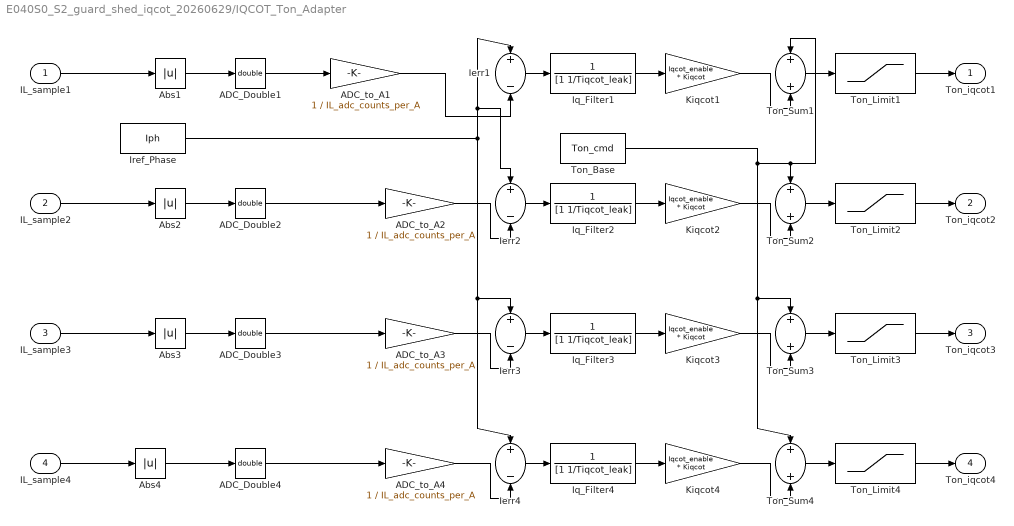
== system E040S0_S2_guard_shed_iqcot_20260629/IQCOT_Ton_Adapter ==
  IL_sample1 : Inport
  IL_sample2 : Inport  Port=2
  IL_sample3 : Inport  Port=3
  IL_sample4 : Inport  Port=4
  ADC_Double{1..4} (4 alike) : DataTypeConversion  OutDataTypeStr=double  SaturateOnIntegerOverflow=off  RndMeth=Floor
  ADC_to_A{1..4} (4 alike) : Gain  Gain=1 / IL_adc_counts_per_A  OutDataTypeStr=double
  Abs{1..4} (4 alike) : Abs  SaturateOnIntegerOverflow=off
  Ierr{1..4} (4 alike) : Sum  Inputs=+-
  Iq_Filter{1..4} (4 alike) : TransferFcn  Numerator=1  Denominator=[1 1/Tiqcot_leak]
  Iref_Phase : Constant  Value=Iph
  Kiqcot{1..4} (4 alike) : Gain  Gain=Iqcot_enable * Kiqcot
  Ton_Base : Constant  Value=Ton_cmd
  Ton_Limit{1..4} (4 alike) : Saturate  UpperLimit=Ton_iq_max  LowerLimit=Ton_iq_min
  Ton_Sum{1..4} (4 alike) : Sum
  Ton_iqcot1 : Outport
  Ton_iqcot2 : Outport  Port=2
  Ton_iqcot3 : Outport  Port=3
  Ton_iqcot4 : Outport  Port=4
  wires:
  IL_sample1/1 -> Abs1/1
  Abs1/1 -> ADC_Double1/1
  ADC_to_A1/1 -> Ierr1/2
  Iref_Phase/1 -> Ierr1/1, Ierr2/1, Ierr3/1, Ierr4/1
  Ierr1/1 -> Iq_Filter1/1
  Iq_Filter1/1 -> Kiqcot1/1
  Kiqcot1/1 -> Ton_Sum1/2
  Ton_Base/1 -> Ton_Sum3/1, Ton_Sum4/1, Ton_Sum1/1, Ton_Sum2/1
  Ton_Sum1/1 -> Ton_Limit1/1
  Ton_Limit1/1 -> Ton_iqcot1/1
  IL_sample2/1 -> Abs2/1
  Abs2/1 -> ADC_Double2/1
  ADC_to_A2/1 -> Ierr2/2
  Ierr2/1 -> Iq_Filter2/1
  Iq_Filter2/1 -> Kiqcot2/1
  Kiqcot2/1 -> Ton_Sum2/2
  Ton_Sum2/1 -> Ton_Limit2/1
  Ton_Limit2/1 -> Ton_iqcot2/1
  IL_sample3/1 -> Abs3/1
  Abs3/1 -> ADC_Double3/1
  ADC_to_A3/1 -> Ierr3/2
  Ierr3/1 -> Iq_Filter3/1
  Iq_Filter3/1 -> Kiqcot3/1
  Kiqcot3/1 -> Ton_Sum3/2
  Ton_Sum3/1 -> Ton_Limit3/1
  Ton_Limit3/1 -> Ton_iqcot3/1
  IL_sample4/1 -> Abs4/1
  Abs4/1 -> ADC_Double4/1
  ADC_to_A4/1 -> Ierr4/2
  Ierr4/1 -> Iq_Filter4/1
  Iq_Filter4/1 -> Kiqcot4/1
  Kiqcot4/1 -> Ton_Sum4/2
  Ton_Sum4/1 -> Ton_Limit4/1
  Ton_Limit4/1 -> Ton_iqcot4/1
  ADC_Double1/1 -> ADC_to_A1/1
  ADC_Double2/1 -> ADC_to_A2/1
  ADC_Double3/1 -> ADC_to_A3/1
  ADC_Double4/1 -> ADC_to_A4/1

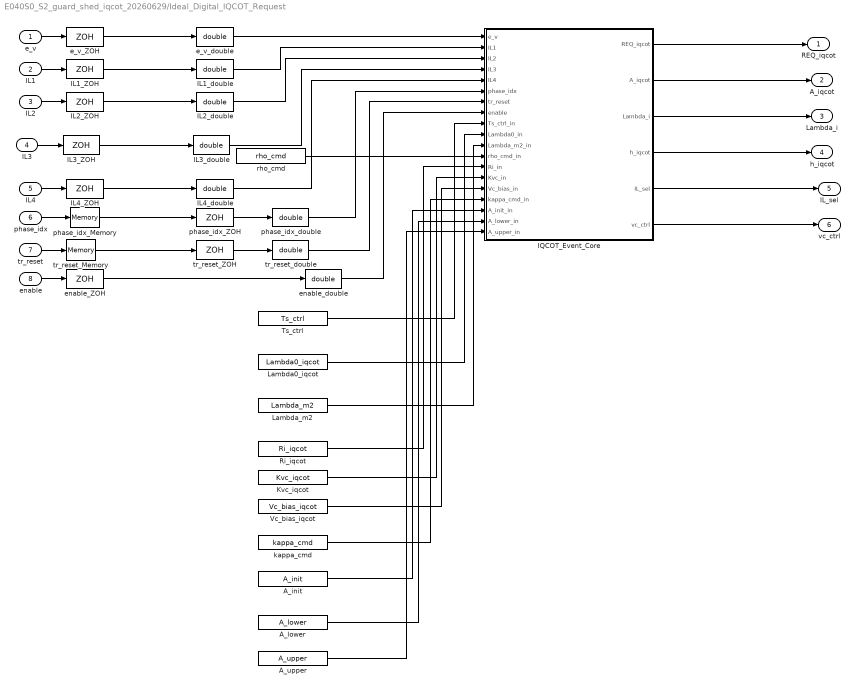
== system E040S0_S2_guard_shed_iqcot_20260629/Ideal_Digital_IQCOT_Request ==
  e_v : Inport
  IL1 : Inport  Port=2
  IL2 : Inport  Port=3
  IL3 : Inport  Port=4
  IL4 : Inport  Port=5
  phase_idx : Inport  Port=6
  tr_reset : Inport  Port=7
  enable : Inport  Port=8
  A_init : Constant  Value=A_init
  A_lower : Constant  Value=A_lower
  A_upper : Constant  Value=A_upper
  IL1_ZOH : ZeroOrderHold  SampleTime=Ts_ctrl
  IL1_double : DataTypeConversion  OutDataTypeStr=double  SaturateOnIntegerOverflow=off  RndMeth=Floor
  IL2_ZOH : ZeroOrderHold  SampleTime=Ts_ctrl
  IL2_double : DataTypeConversion  OutDataTypeStr=double  SaturateOnIntegerOverflow=off  RndMeth=Floor
  IL3_ZOH : ZeroOrderHold  SampleTime=Ts_ctrl
  IL3_double : DataTypeConversion  OutDataTypeStr=double  SaturateOnIntegerOverflow=off  RndMeth=Floor
  IL4_ZOH : ZeroOrderHold  SampleTime=Ts_ctrl
  IL4_double : DataTypeConversion  OutDataTypeStr=double  SaturateOnIntegerOverflow=off  RndMeth=Floor
  IQCOT_Event_Core : MATLAB Function  TreatAsAtomicUnit=on
  Kvc_iqcot : Constant  Value=Kvc_iqcot
  Lambda0_iqcot : Constant  Value=Lambda0_iqcot
  Lambda_m2 : Constant  Value=Lambda_m2
  Ri_iqcot : Constant  Value=Ri_iqcot
  Ts_ctrl : Constant  Value=Ts_ctrl
  Vc_bias_iqcot : Constant  Value=Vc_bias_iqcot
  e_v_ZOH : ZeroOrderHold  SampleTime=Ts_ctrl
  e_v_double : DataTypeConversion  OutDataTypeStr=double  SaturateOnIntegerOverflow=off  RndMeth=Floor
  enable_ZOH : ZeroOrderHold  SampleTime=Ts_ctrl
  enable_double : DataTypeConversion  OutDataTypeStr=double  SaturateOnIntegerOverflow=off  RndMeth=Floor
  kappa_cmd : Constant  Value=kappa_cmd
  phase_idx_Memory : Memory
  phase_idx_ZOH : ZeroOrderHold  SampleTime=Ts_ctrl
  phase_idx_double : DataTypeConversion  OutDataTypeStr=double  SaturateOnIntegerOverflow=off  RndMeth=Floor
  rho_cmd : Constant  Value=rho_cmd
  tr_reset_Memory : Memory
  tr_reset_ZOH : ZeroOrderHold  SampleTime=Ts_ctrl
  tr_reset_double : DataTypeConversion  OutDataTypeStr=double  SaturateOnIntegerOverflow=off  RndMeth=Floor
  REQ_iqcot : Outport
  A_iqcot : Outport  Port=2
  Lambda_i : Outport  Port=3
  h_iqcot : Outport  Port=4
  IL_sel : Outport  Port=5
  vc_ctrl : Outport  Port=6
  wires:
  e_v/1 -> e_v_ZOH/1
  e_v_ZOH/1 -> e_v_double/1
  IL1/1 -> IL1_ZOH/1
  IL1_ZOH/1 -> IL1_double/1
  IL2/1 -> IL2_ZOH/1
  IL2_ZOH/1 -> IL2_double/1
  IL3/1 -> IL3_ZOH/1
  IL3_ZOH/1 -> IL3_double/1
  IL4/1 -> IL4_ZOH/1
  IL4_ZOH/1 -> IL4_double/1
  phase_idx/1 -> phase_idx_Memory/1
  phase_idx_Memory/1 -> phase_idx_ZOH/1
  phase_idx_ZOH/1 -> phase_idx_double/1
  tr_reset/1 -> tr_reset_Memory/1
  tr_reset_Memory/1 -> tr_reset_ZOH/1
  tr_reset_ZOH/1 -> tr_reset_double/1
  enable/1 -> enable_ZOH/1
  enable_ZOH/1 -> enable_double/1
  e_v_double/1 -> IQCOT_Event_Core/1(e_v)
  IL1_double/1 -> IQCOT_Event_Core/2(IL1)
  IL2_double/1 -> IQCOT_Event_Core/3(IL2)
  IL3_double/1 -> IQCOT_Event_Core/4(IL3)
  IL4_double/1 -> IQCOT_Event_Core/5(IL4)
  phase_idx_double/1 -> IQCOT_Event_Core/6(phase_idx)
  tr_reset_double/1 -> IQCOT_Event_Core/7(tr_reset)
  enable_double/1 -> IQCOT_Event_Core/8(enable)
  Ts_ctrl/1 -> IQCOT_Event_Core/9(Ts_ctrl_in)
  Lambda0_iqcot/1 -> IQCOT_Event_Core/10(Lambda0_in)
  Lambda_m2/1 -> IQCOT_Event_Core/11(Lambda_m2_in)
  rho_cmd/1 -> IQCOT_Event_Core/12(rho_cmd_in)
  Ri_iqcot/1 -> IQCOT_Event_Core/13(Ri_in)
  Kvc_iqcot/1 -> IQCOT_Event_Core/14(Kvc_in)
  Vc_bias_iqcot/1 -> IQCOT_Event_Core/15(Vc_bias_in)
  kappa_cmd/1 -> IQCOT_Event_Core/16(kappa_cmd_in)
  A_init/1 -> IQCOT_Event_Core/17(A_init_in)
  A_lower/1 -> IQCOT_Event_Core/18(A_lower_in)
  A_upper/1 -> IQCOT_Event_Core/19(A_upper_in)
  IQCOT_Event_Core/1(REQ_iqcot) -> REQ_iqcot/1
  IQCOT_Event_Core/2(A_iqcot) -> A_iqcot/1
  IQCOT_Event_Core/3(Lambda_i) -> Lambda_i/1
  IQCOT_Event_Core/4(h_iqcot) -> h_iqcot/1
  IQCOT_Event_Core/5(IL_sel) -> IL_sel/1
  IQCOT_Event_Core/6(vc_ctrl) -> vc_ctrl/1

== system E040S0_S2_guard_shed_iqcot_20260629/OnDelay ==
  u : Inport
  Compare To Constant : simulink/Logic and Bit Operations/Compare To Constant  relop=>=  const=Tdead  OutDataTypeStr=boolean
  Data Type Conversion : DataTypeConversion  OutDataTypeStr=double  SaturateOnIntegerOverflow=off  RndMeth=Floor
  Integrator : Integrator  ExternalReset=level
  Logical Operator : Logic  Operator=NOT  AllPortsSameDT=off  OutDataTypeStr=boolean
  y : Outport
  wires:
  u/1 -> Data Type Conversion/1, Logical Operator/1
  Logical Operator/1 -> Integrator/2
  Data Type Conversion/1 -> Integrator/1
  Integrator/1 -> Compare To Constant/1
  Compare To Constant/1 -> y/1

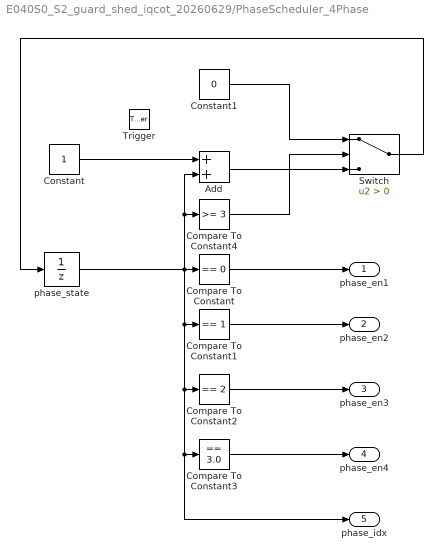
== system E040S0_S2_guard_shed_iqcot_20260629/PhaseScheduler_4Phase ==
  Trigger : TriggerPort  VariantControl=(inherit)
  Add : Sum
  Compare To Constant : simulink/Logic and Bit Operations/Compare To Constant  relop===  const=0  OutDataTypeStr=boolean
  Compare To Constant1 : simulink/Logic and Bit Operations/Compare To Constant  relop===  const=1  OutDataTypeStr=boolean
  Compare To Constant2 : simulink/Logic and Bit Operations/Compare To Constant  relop===  const=2  OutDataTypeStr=boolean
  Compare To Constant3 : simulink/Logic and Bit Operations/Compare To Constant  relop===  const=3.0  OutDataTypeStr=boolean
  Compare To Constant4 : simulink/Logic and Bit Operations/Compare To Constant  relop=>=  const=3  OutDataTypeStr=boolean
  Constant : Constant
  Constant1 : Constant  Value=0
  Switch : Switch  Criteria=u2 > Threshold  SaturateOnIntegerOverflow=off  InputSameDT=off
  phase_state : UnitDelay  SampleTime=-1  HasFrameUpgradeWarning=on
  phase_en1 : Outport
  phase_en2 : Outport  Port=2
  phase_en3 : Outport  Port=3
  phase_en4 : Outport  Port=4
  phase_idx : Outport  Port=5
  wires:
  phase_state/1 -> phase_idx/1, Compare To Constant3/1, Compare To Constant2/1, Compare To Constant1/1, Compare To Constant/1, Compare To Constant4/1, Add/2
  Compare To Constant/1 -> phase_en1/1
  Compare To Constant1/1 -> phase_en2/1
  Compare To Constant2/1 -> phase_en3/1
  Compare To Constant3/1 -> phase_en4/1
  Constant/1 -> Add/1
  Add/1 -> Switch/3
  Compare To Constant4/1 -> Switch/2
  Constant1/1 -> Switch/1
  Switch/1 -> phase_state/1

== system E040S0_S2_guard_shed_iqcot_20260629/GateDriver_1Phase1/OnDelay ==
  u : Inport
  Compare To Constant : simulink/Logic and Bit Operations/Compare To Constant  relop=>=  const=Tdead  OutDataTypeStr=boolean
  Data Type Conversion : DataTypeConversion  OutDataTypeStr=double  SaturateOnIntegerOverflow=off  RndMeth=Floor
  Integrator : Integrator  ExternalReset=level
  Logical Operator : Logic  Operator=NOT  AllPortsSameDT=off  OutDataTypeStr=boolean
  y : Outport
  wires:
  u/1 -> Data Type Conversion/1, Logical Operator/1
  Logical Operator/1 -> Integrator/2
  Data Type Conversion/1 -> Integrator/1
  Integrator/1 -> Compare To Constant/1
  Compare To Constant/1 -> y/1

== system E040S0_S2_guard_shed_iqcot_20260629/GateDriver_1Phase1/OnDelay1 ==
  u : Inport
  Compare To Constant : simulink/Logic and Bit Operations/Compare To Constant  relop=>=  const=Tdead  OutDataTypeStr=boolean
  Data Type Conversion : DataTypeConversion  OutDataTypeStr=double  SaturateOnIntegerOverflow=off  RndMeth=Floor
  Integrator : Integrator  ExternalReset=level
  Logical Operator : Logic  Operator=NOT  AllPortsSameDT=off  OutDataTypeStr=boolean
  y : Outport
  wires:
  u/1 -> Data Type Conversion/1, Logical Operator/1
  Logical Operator/1 -> Integrator/2
  Data Type Conversion/1 -> Integrator/1
  Integrator/1 -> Compare To Constant/1
  Compare To Constant/1 -> y/1

== system E040S0_S2_guard_shed_iqcot_20260629/GateDriver_1Phase2/OnDelay ==
  u : Inport
  Compare To Constant : simulink/Logic and Bit Operations/Compare To Constant  relop=>=  const=Tdead  OutDataTypeStr=boolean
  Data Type Conversion : DataTypeConversion  OutDataTypeStr=double  SaturateOnIntegerOverflow=off  RndMeth=Floor
  Integrator : Integrator  ExternalReset=level
  Logical Operator : Logic  Operator=NOT  AllPortsSameDT=off  OutDataTypeStr=boolean
  y : Outport
  wires:
  u/1 -> Data Type Conversion/1, Logical Operator/1
  Logical Operator/1 -> Integrator/2
  Data Type Conversion/1 -> Integrator/1
  Integrator/1 -> Compare To Constant/1
  Compare To Constant/1 -> y/1

== system E040S0_S2_guard_shed_iqcot_20260629/GateDriver_1Phase2/OnDelay1 ==
  u : Inport
  Compare To Constant : simulink/Logic and Bit Operations/Compare To Constant  relop=>=  const=Tdead  OutDataTypeStr=boolean
  Data Type Conversion : DataTypeConversion  OutDataTypeStr=double  SaturateOnIntegerOverflow=off  RndMeth=Floor
  Integrator : Integrator  ExternalReset=level
  Logical Operator : Logic  Operator=NOT  AllPortsSameDT=off  OutDataTypeStr=boolean
  y : Outport
  wires:
  u/1 -> Data Type Conversion/1, Logical Operator/1
  Logical Operator/1 -> Integrator/2
  Data Type Conversion/1 -> Integrator/1
  Integrator/1 -> Compare To Constant/1
  Compare To Constant/1 -> y/1

== system E040S0_S2_guard_shed_iqcot_20260629/GateDriver_1Phase3/OnDelay ==
  u : Inport
  Compare To Constant : simulink/Logic and Bit Operations/Compare To Constant  relop=>=  const=Tdead  OutDataTypeStr=boolean
  Data Type Conversion : DataTypeConversion  OutDataTypeStr=double  SaturateOnIntegerOverflow=off  RndMeth=Floor
  Integrator : Integrator  ExternalReset=level
  Logical Operator : Logic  Operator=NOT  AllPortsSameDT=off  OutDataTypeStr=boolean
  y : Outport
  wires:
  u/1 -> Data Type Conversion/1, Logical Operator/1
  Logical Operator/1 -> Integrator/2
  Data Type Conversion/1 -> Integrator/1
  Integrator/1 -> Compare To Constant/1
  Compare To Constant/1 -> y/1
